simulink model "Senorless"  (R2023a)
settings: Solver=FixedStepDiscrete  StartTime=0.0  StopTime=2  FixedStep=1/FOC_FRQ  RelTol=1e-3
values from neighbouring files (symbols this model uses):
  ADC_REF = 3.6    [Senorless.sldd]
  ADC_SAMPLE_MAX = 32767.0    [Senorless.sldd]
  AMP_GAIN = 32.0    [Senorless.sldd]
  CURR_INPUT = 3276.0    [Senorless.sldd]
  CURR_KI = 380.0    [Senorless.sldd]
  CURR_KP = 0.04    [Senorless.sldd]
  CURR_LIMIT = 1.1    [Senorless.sldd]
  CURR_OVER = 34.0    [Senorless.sldd]
  CURR_POINT_GAIN = 7.0    [Senorless.sldd]
  CURR_STEP = 32760.0    [Senorless.sldd]
  CURR_UNDER = 0.03    [Senorless.sldd]
  CURR_WIDTH = 250.0    [Senorless.sldd]
  FOC_FRQ = 36000.0    [Senorless.sldd]
  GAMMA = 32767.0    [Senorless.sldd]
  HFI_ID = 2.125    [Senorless.sldd]
  IMAX = 34.0    [Senorless.sldd]
  LPF_FRQ = 300.0    [Senorless.sldd]
  MOTOR_DAMPER = 8.3E-7    [Senorless.sldd]
  MOTOR_FLUX = 0.0012713112    [Senorless.sldd]
  MOTOR_INERTIA = 1.02E-6    [Senorless.sldd]
  MOTOR_LS = 1.8E-5    [Senorless.sldd]
  MOTOR_PN = 7.0    [Senorless.sldd]
  MOTOR_RS = 0.065    [Senorless.sldd]
  NS_COMP_UD = 0.531    [Senorless.sldd]
  PLL_LIMIT = 0.95    [Senorless.sldd]
  PLL_WIDTH = 500.0    [Senorless.sldd]
  PWM_FRQ = 96000000.0    [Senorless.sldd]
  RS_HUNT = 0.002    [Senorless.sldd]
  SMOK_FRQ = 1200.0    [Senorless.sldd]
  SPD_LIMIT = 0.8    [Senorless.sldd]
  SPD_LPF_LEVEL = 15.0    [Senorless.sldd]
  SPD_MAX = 8100.0    [Senorless.sldd]
  SPD_MIN = -8100.0    [Senorless.sldd]
  SPD_REDUCE = 380.0    [Senorless.sldd]
  SPD_STEP = 3.0    [Senorless.sldd]
  SPD_WIDTH = 10.0    [Senorless.sldd]
  TS_POINT_GAIN = 10.0    [Senorless.sldd]
  UDC = 17.0    [Senorless.sldd]
  UDC_GAIN = 21.0    [Senorless.sldd]
  UDC_POINT_GAIN = 10.0    [Senorless.sldd]
undefined symbols (not defined in the file or in its folder): curr_q_ki, curr_q_kp, DiscIntNeverNeededParam, magnitude, PLL_LPF_LEVEL, Udc
libraries: simulink x20, slpidlib x5, mcbcontrolslib x4, mcbplantlib x1, autolibpmsminterior x1, autolibpmsmexterior x1, spspowerguiLib x1
(part 5 of 7)

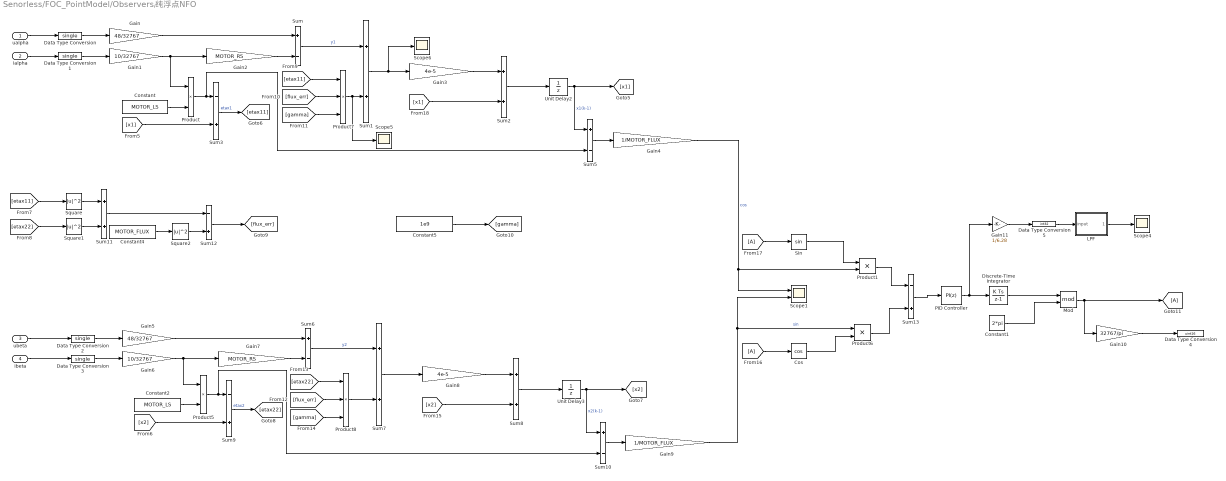
== system Senorless/FOC_PointModel/Observers/纯浮点NFO ==
  ualpha : Inport
  ialpha : Inport  Port=2
  ubeta : Inport  Port=3
  ibeta : Inport  Port=4
  Constant : Constant  Value=MOTOR_LS
  Constant1 : Constant  Value=2*pi  OutDataTypeStr=single
  Constant2 : Constant  Value=MOTOR_LS
  Constant4 : Constant  Value=MOTOR_FLUX
  Constant5 : Constant  Value=1e9  OutDataTypeStr=single
  Cos : Trigonometry  Operator=cos
  Data Type Conversion{,1..3} (4 alike) : DataTypeConversion  OutDataTypeStr=single  SaturateOnIntegerOverflow=off  RndMeth=Floor
  Data Type Conversion4 : DataTypeConversion  OutDataTypeStr=uint16  SaturateOnIntegerOverflow=off  RndMeth=Floor
  Data Type Conversion5 : DataTypeConversion  OutDataTypeStr=int32  SaturateOnIntegerOverflow=off  RndMeth=Floor
  Discrete-Time Integrator : DiscreteIntegrator  SampleTime=-1  ICPrevOutput=DiscIntNeverNeededParam  ICPrevScaledInput=DiscIntNeverNeededParam
  From16 : From
  From17 : From
  Gain : Gain  Gain=48/32767
  Gain1 : Gain  Gain=10/32767
  Gain10 : Gain  Gain=32767/pi
  Gain11 : Gain  Gain=1/6.28
  Gain2 : Gain  Gain=MOTOR_RS
  Gain3 : Gain  Gain=4e-5  OutDataTypeStr=single
  Gain4 : Gain  Gain=1/MOTOR_FLUX
  Gain5 : Gain  Gain=48/32767
  Gain6 : Gain  Gain=10/32767
  Gain7 : Gain  Gain=MOTOR_RS
  Gain8 : Gain  Gain=4e-5  OutDataTypeStr=single
  Gain9 : Gain  Gain=1/MOTOR_FLUX
  Goto11 : Goto
  LPF : Subsystem  TreatAsAtomicUnit=on
  Mod : Math  Operator=mod
  PID Controller : slpidlib/PID Controller  Controller=PI  Form=Parallel  TimeDomain=Discrete-time  UseExternalTs=off  SampleTime=-1  IntegratorMethod=Forward Euler  FilterMethod=Forward Euler  ControllerParametersSource=internal  P=2*800  I=800*800  UseKiTs=off  D=0  N=100  UseFilter=on  TunerSelectOption=Transfer Function Based (PID Tuner App)  InitialConditionSource=internal  InitialConditionForIntegrator=0  InitialConditionForFilter=0  DifferentiatorICPrevScaledInput=0  ExternalReset=none  TrackingMode=off  Kt=1  LimitOutput=off  SatLimitsSource=internal  UpperSaturationLimit=inf  LowerSaturationLimit=-inf  LinearizeAsGain=on  AntiWindupMode=none  Kb=1  LimitIntegrator=off  UpperIntegratorSaturationLimit=inf  LowerIntegratorSaturationLimit=-inf  POutMin=[]  POutMax=[]  IOutMin=[]  IOutMax=[]  DOutMin=[]  DOutMax=[]  NOutMin=[]  NOutMax=[]  SumOutMin=[]  SumOutMax=[]  SaturationOutMin=[]  SaturationOutMax=[]  PParamMin=[]  PParamMax=[]  IParamMin=[]  IParamMax=[]  DParamMin=[]  DParamMax=[]  NParamMin=[]  NParamMax=[]  KbParamMin=[]  KbParamMax=[]  KtParamMin=[]  KtParamMax=[]  KbOutMin=[]  KbOutMax=[]  KtOutMin=[]  KtOutMax=[]  IntegratorOutMin=[]  IntegratorOutMax=[]  FilterOutMin=[]  FilterOutMax=[]  SumI1OutMin=[]  SumI1OutMax=[]  SumI2OutMin=[]  SumI2OutMax=[]  SumI3OutMin=[]  SumI3OutMax=[]  SumI4OutMin=[]  SumI4OutMax=[]  SumDOutMin=[]  SumDOutMax=[]  DifferentiatorOutMin=[]  DifferentiatorOutMax=[]  FilterDiffOutCoefMin=[]  FilterDiffOutCoefMax=[]  ReciprocalOutMin=[]  ReciprocalOutMax=[]  SumDenOutMin=[]  SumDenOutMax=[]  SumNumOutMin=[]  SumNumOutMax=[]  DivideOutMin=[]  DivideOutMax=[]  UdiffTsProdOutMin=[]  UdiffTsProdOutMax=[]  NTsProdOutMin=[]  NTsProdOutMax=[]  UintegralTsProdOutMin=[]  UintegralTsProdOutMax=[]  UngainTsProdOutMin=[]  UngainTsProdOutMax=[]  ClampingZeroOutDataTypeStr=Inherit: Inherit via back propagation  ClampingZeroOutMin=[]  ClampingZeroOutMax=[]  FilterDenConstantOutDataTypeStr=Inherit: Inherit via back propagation  FilterDenConstantOutMin=[]  FilterDenConstantOutMax=[]  PCopyOutDataTypeStr=Inherit: Inherit via back propagation  PCopyOutMin=[]  PCopyOutMax=[]  NCopyOutDataTypeStr=Inherit: Inherit via back propagation  NCopyOutMin=[]  NCopyOutMax=[]  IntegratorContinuousStateAttributes=''  IntegratorStateMustResolveToSignalObject=off  IntegratorRTWStateStorageClass=Auto  FilterContinuousStateAttributes=''  FilterStateMustResolveToSignalObject=off  FilterRTWStateStorageClass=Auto  ParallelPVariant=InternalParameters  IdealPVariant=Disabled  IVariant=InternalParameters  DVariant=Disabled  IntegratorVariant=Discrete  SatVariant=Disabled  AWVariant=Passthrough  PCopyVariant=Disabled  TRVariant=Disabled  FdbkBlocksVariant=Forward  IdealPFdbkVariant=Disabled  SatFdbkVariant=Disabled  DerivativeFilterVariant=Disabled  NVariant=Disabled  NCopyVariant=Disabled_SignalSpec  FilterICVariant=Disabled  IntegratorICVariant=InternalICs  ExternalResetVariant=Disabled  TRSumVariant=Passthrough  SumFdbkVariant=Disabled  SumVariant=Sum_PI  TsampFilterVariant=InternalTs  TsampNgainVariant=Passthrough  TsampIntegralVariant=Disabled_SignalSpec  ExternalSaturationOutDataTypeStr=Inherit: Same as second input
  Product{,1,5..6} (4 alike) : Product
  Product7 : Product  Inputs=3
  Product8 : Product  Inputs=3
  Scope1 : Scope  NumInputPorts=2
  Scope4 : Scope
  Scope5 : Scope
  Scope6 : Scope
  Sin : Trigonometry
  Square : Math  Operator=magnitude^2  OutputSignalType=real
  Square1 : Math  Operator=magnitude^2  OutputSignalType=real
  Square2 : Math  Operator=magnitude^2  OutputSignalType=real
  Sum{,5..6,10} (4 alike) : Sum  Inputs=+-
  Sum{1..2,7..8,11} (5 alike) : Sum
  Sum{3,9,12..13} (4 alike) : Sum  Inputs=-+
  Unit Delay2 : UnitDelay  SampleTime=-1  HasFrameUpgradeWarning=on
  Unit Delay3 : UnitDelay  SampleTime=-1  HasFrameUpgradeWarning=on
  wires:
  Gain8/1 -> Sum8/1
  Constant2/1 -> Product5/2
  Sum/1 -> Sum1/1  "y1"
  Sum2/1 -> Unit Delay2/1
  Sum10/1 -> Gain9/1
  Gain4/1 -> Scope1/1, Product1/2  "cos"
  [x1] -> Sum2/2
  ibeta/1 -> Data Type Conversion3/1
  ubeta/1 -> Data Type Conversion2/1
  [etax22] -> Square1/1
  Data Type Conversion/1 -> Gain/1
  [etax11] -> Square/1
  Sum9/1 -> [etax22]  "etax2"
  Gain/1 -> Sum/1
  Product5/1 -> Sum10/2, Sum9/1
  Square2/1 -> Sum12/2
  Product1/1 -> Sum13/1
  Gain5/1 -> Sum6/1
  Sum1/1 -> Scope6/1, Gain3/1
  Data Type Conversion3/1 -> Gain6/1
  Sum8/1 -> Unit Delay3/1
  [flux_err] -> Product8/2
  Sum5/1 -> Gain4/1
  PID Controller/1 -> Gain11/1, Discrete-Time Integrator/1
  Cos/1 -> Product6/2
  [etax22] -> Product8/1
  [gamma] -> Product7/3
  Square1/1 -> Sum11/2
  [x1] -> Sum3/2
  Constant/1 -> Product/2
  Product7/1 -> Scope5/1, Sum1/2
  Sum13/1 -> PID Controller/1
  Square/1 -> Sum11/1
  Sum6/1 -> Sum7/1  "y2"
  Product8/1 -> Sum7/2
  Discrete-Time Integrator/1 -> Mod/1
  [flux_err] -> Product7/2
  Constant5/1 -> [gamma]
  Constant4/1 -> Square2/1
  Sum12/1 -> [flux_err]
  [gamma] -> Product8/3
  Sum3/1 -> [etax11]  "etax1"
  Gain9/1 -> Scope1/2, Product6/1  "sin"
  [etax11] -> Product7/1
  Gain7/1 -> Sum6/2
  Gain1/1 -> Product/1, Gain2/1
  Gain10/1 -> Data Type Conversion4/1
  ialpha/1 -> Data Type Conversion1/1
  Gain6/1 -> Gain7/1, Product5/1
  Gain3/1 -> Sum2/1
  Sin/1 -> Product1/1
  Product6/1 -> Sum13/2
  Sum11/1 -> Sum12/1
  From17/1 -> Sin/1
  Data Type Conversion1/1 -> Gain1/1
  Gain11/1 -> Data Type Conversion5/1
  Mod/1 -> Gain10/1, Goto11/1
  From16/1 -> Cos/1
  Constant1/1 -> Mod/2
  [x2] -> Sum8/2
  Gain2/1 -> Sum/2
  [x2] -> Sum9/2
  Data Type Conversion2/1 -> Gain5/1
  Sum7/1 -> Gain8/1
  Unit Delay3/1 -> Sum10/1, [x2]  "x2(k-1)"
  Unit Delay2/1 -> Sum5/1, [x1]  "x1(k-1)"
  Product/1 -> Sum5/2, Sum3/1
  LPF/1(output) -> Scope4/1
  Data Type Conversion5/1 -> LPF/1(input)
  ualpha/1 -> Data Type Conversion/1

== system Senorless/FOC_PointModel/Park/滤波器 ==
  input : Inport
  Constant13 : Constant  Value=2*pi*250  OutDataTypeStr=int32
  Gain : Gain  Gain=1.414*32767  ParamDataTypeStr=int32  OutDataTypeStr=int32  RndMeth=Zero
  Gain1 : Gain  Gain=0.707*32767  ParamDataTypeStr=int32  OutDataTypeStr=int32  RndMeth=Zero
  Product : Product  OutDataTypeStr=int32  RndMeth=Zero
  Product1 : Product  OutDataTypeStr=int32  RndMeth=Zero
  Scope : Scope  NumInputPorts=2
  Shift Arithmetic : ArithShift  BitShiftNumber=15
  Shift Arithmetic1 : ArithShift  BitShiftNumber=15
  Sum5 : Sum  Inputs=-+|  AccumDataTypeStr=int32  OutDataTypeStr=int32  RndMeth=Zero
  Sum8 : Sum  Inputs=|+-  AccumDataTypeStr=int32  OutDataTypeStr=int32  RndMeth=Zero
  Unit Delay : UnitDelay  SampleTime=-1  HasFrameUpgradeWarning=on
  input1 : InportShadow
  积分器4 : Subsystem
      settings: MinAlgLoopOccurrences=on
  积分器5 : Subsystem
      settings: MinAlgLoopOccurrences=on
  output : Outport
  wires:
  Constant13/1 -> Product/2, Product1/1
  Product/1 -> 积分器4/1(input)
  Product1/1 -> 积分器5/1(input)
  Sum8/1 -> Product/1
  input1/1 -> Scope/2
  积分器4/1(output) -> Unit Delay/1
  Unit Delay/1 -> Sum5/1, Product1/2
  Gain/1 -> Shift Arithmetic/1
  Gain1/1 -> Shift Arithmetic1/1
  积分器5/1(output) -> Gain1/1, Sum8/2
  Shift Arithmetic1/1 -> Scope/1, output/1
  input/1 -> Sum5/2
  Sum5/1 -> Gain/1
  Shift Arithmetic/1 -> Sum8/1

== system Senorless/FOC_PointModel/SVPWM/AntiClark ==
  note: Va = Valpha;
      | Vb = Valpha*(-1/2)+Vbeta*sqrt(3)/2
      | Vc = Valpha*(-1/2)-Vbeta*sqrt(3)/2
  Valpha : Inport
  Vbeta : Inport  Port=2
  Gain1 : Gain  Gain=32767*sqrt(3)/2  ParamDataTypeStr=int16  OutDataTypeStr=int32  RndMeth=Zero
  Shift Arithmetic : ArithShift  BitShiftNumber=15
  Shift Arithmetic1 : ArithShift  BitShiftNumber=1
  Sum : Sum  Inputs=|-+  RndMeth=Zero
  Sum1 : Sum  Inputs=--|  RndMeth=Zero
  Va : Outport
  Vb : Outport  Port=2
  Vc : Outport  Port=3
  wires:
  Vbeta/1 -> Gain1/1
  Shift Arithmetic1/1 -> Sum1/2, Sum/1
  Sum/1 -> Vb/1
  Gain1/1 -> Shift Arithmetic/1
  Sum1/1 -> Vc/1
  Shift Arithmetic/1 -> Sum1/1, Sum/2
  Valpha/1 -> Va/1, Shift Arithmetic1/1

== system Senorless/FOC_PointModel/SVPWM/ei_t ==
  note: V0 = -1/2(Vmax+Vmin)
  Vabc : Inport
  Min : MinMax  RndMeth=Zero
  Min1 : MinMax  Function=max  RndMeth=Zero
  Shift Arithmetic : ArithShift  BitShiftNumber=1
  Sum : Sum  OutDataTypeStr=int32  RndMeth=Zero
  Unary Minus : UnaryMinus
  ei_t : Outport
  wires:
  Min/1 -> Sum/1
  Sum/1 -> Shift Arithmetic/1
  Min1/1 -> Sum/2
  Shift Arithmetic/1 -> Unary Minus/1
  Unary Minus/1 -> ei_t/1
  Vabc/1 -> Min1/1, Min/1

== system Senorless/FOC_PointModel/idq_Controller/PI Controller ==
  input : Inport
  Kp : Inport  Port=2
  Ki : Inport  Port=3
  Data Store Read3 : DataStoreRead  DataStoreName=Curr_Limit  IndexOptions=Index vector (dialog)  Indices=1  OutputSizes=1
  Gain : Gain  Gain=-1  OutDataTypeStr=int32  RndMeth=Zero
  Product2 : Product  OutDataTypeStr=int32  RndMeth=Zero
  Saturation Dynamic2 : simulink/Discontinuities/Saturation Dynamic  OutMin=[]  OutMax=[]  OutDataTypeStr=Inherit: Same as second input  OutDataType=fixdt(1, 16)  OutScaling=2^-10  RndMeth=Zero  DoSatur=off
  Scope : Scope  NumInputPorts=2
  Sum : Sum  OutDataTypeStr=int32  RndMeth=Zero
  input1 : InportShadow
  积分器 : Subsystem
      settings: MinAlgLoopOccurrences=on
  output : Outport  OutputWhenDisabled=reset  InitialOutput=int32(0)
  wires:
  input/1 -> Product2/1
  Kp/1 -> Product2/2
  Ki/1 -> 积分器/1(Ki)
  input1/1 -> 积分器/2(input)
  Product2/1 -> Scope/1, Sum/1
  积分器/1(output) -> Sum/2, Scope/2
  Sum/1 -> Saturation Dynamic2/2
  Saturation Dynamic2/1 -> output/1
  Data Store Read3/1 -> [limit]
  [limit] -> Gain/1
  Gain/1 -> Saturation Dynamic2/3
  [limit] -> Saturation Dynamic2/1

== system Senorless/FOC_PointModel/idq_Controller/PI Controller1 ==
  Ki : Inport
  Kp : Inport  Port=2
  input : Inport  Port=3
  Data Store Read3 : DataStoreRead  DataStoreName=Curr_Limit  IndexOptions=Index vector (dialog)  Indices=1  OutputSizes=1
  Gain : Gain  Gain=-1  OutDataTypeStr=int32  RndMeth=Zero
  Product2 : Product  OutDataTypeStr=int32  RndMeth=Zero
  Saturation Dynamic2 : simulink/Discontinuities/Saturation Dynamic  OutMin=[]  OutMax=[]  OutDataTypeStr=Inherit: Same as second input  OutDataType=fixdt(1, 16)  OutScaling=2^-10  RndMeth=Zero  DoSatur=off
  Scope : Scope  NumInputPorts=2
  Sum : Sum  OutDataTypeStr=int32  RndMeth=Zero
  input1 : InportShadow  Port=3
  积分器 : Subsystem
      settings: MinAlgLoopOccurrences=on
  output : Outport  OutputWhenDisabled=reset  InitialOutput=int32(0)
  wires:
  [limit] -> Saturation Dynamic2/1
  Gain/1 -> Saturation Dynamic2/3
  [limit] -> Gain/1
  Data Store Read3/1 -> [limit]
  Sum/1 -> Saturation Dynamic2/2
  积分器/1(output) -> Scope/2, Sum/2
  Product2/1 -> Sum/1, Scope/1
  input1/1 -> 积分器/2(input)
  Ki/1 -> 积分器/1(Ki)
  Kp/1 -> Product2/2
  input/1 -> Product2/1
  Saturation Dynamic2/1 -> output/1

== system Senorless/FOC_PointModel/idq_Controller/PI Controller2 ==
  input : Inport
  Kp : Inport  Port=2
  Ki : Inport  Port=3
  Reset : Inport  Port=4
  Xo : Inport  Port=5
  Action Port : ActionPort  InitializeStates=reset  ActionPortLabel=if(u1 > 0)
  Data Store Read3 : DataStoreRead  DataStoreName=Curr_Limit  IndexOptions=Index vector (dialog)  Indices=1  OutputSizes=1
  Gain : Gain  Gain=-1  OutDataTypeStr=int32  RndMeth=Zero
  MATLAB Function : MATLAB Function  TreatAsAtomicUnit=on
  Product2 : Product  OutDataTypeStr=int32  RndMeth=Zero
  Scope : Scope  NumInputPorts=2
  Sum : Sum  OutDataTypeStr=int32  RndMeth=Zero
  input1 : InportShadow
  积分器/双边沿初始化 : Subsystem
      settings: MinAlgLoopOccurrences=on
  output : Outport
  wires:
  [limit] -> MATLAB Function/2(up), Gain/1
  Gain/1 -> MATLAB Function/3(low)
  Data Store Read3/1 -> [limit]
  MATLAB Function/1(out) -> output/1
  Sum/1 -> MATLAB Function/1(in)
  积分器/双边沿初始化/1(output) -> Scope/2, Sum/2
  Product2/1 -> Sum/1, Scope/1
  input1/1 -> 积分器/双边沿初始化/2(input)
  Reset/1 -> 积分器/双边沿初始化/4(Reset)
  Xo/1 -> 积分器/双边沿初始化/3(Xo)
  Ki/1 -> 积分器/双边沿初始化/1(Ki)
  Kp/1 -> Product2/2
  input/1 -> Product2/1

== system Senorless/FOC_PointModel/idq_Controller/Subsystem ==
  Ud : Inport
  Uq : Inport  Port=2
  Constant : Constant  Value=16384*0.9  OutDataTypeStr=int16
  Data Type Conversion5 : DataTypeConversion  OutDataTypeStr=int16  SaturateOnIntegerOverflow=off
  Data Type Conversion6 : DataTypeConversion  OutDataTypeStr=int16  SaturateOnIntegerOverflow=off
  Scope : Scope
  Shift Arithmetic7 : ArithShift  BitShiftNumber=-0
  Sqrt1 : Sqrt  OutputSignalType=real  OutDataTypeStr=int16  RndMeth=Zero  IntermediateResultsDataTypeStr=int32
  Square2 : Math  Operator=square  OutputSignalType=real  OutDataTypeStr=int32  RndMeth=Zero
      settings: LockScale=on
  Square3 : Math  Operator=square  OutDataTypeStr=int32  RndMeth=Zero
      settings: LockScale=on
  Sum11 : Sum  AccumDataTypeStr=int32  OutDataTypeStr=int32
  Sum12 : Sum  Inputs=|-+
  Unit Delay5 : UnitDelay  SampleTime=-1  HasFrameUpgradeWarning=on
  Wrap To Zero1 : simulink/Discontinuities/Wrap To Zero  Threshold=int16(0)
  -Id : Outport
  wires:
  Data Type Conversion5/1 -> Square2/1
  Wrap To Zero1/1 -> Shift Arithmetic7/1
  Sum11/1 -> Sqrt1/1
  Sqrt1/1 -> Scope/1, Sum12/1
  Data Type Conversion6/1 -> Square3/1
  Square2/1 -> Sum11/1
  Sum12/1 -> Wrap To Zero1/1
  Constant/1 -> Sum12/2
  Uq/1 -> Data Type Conversion6/1
  Square3/1 -> Sum11/2
  Ud/1 -> Data Type Conversion5/1
  Shift Arithmetic7/1 -> Unit Delay5/1
  Unit Delay5/1 -> -Id/1

== system Senorless/FOC_PointModel/标志位/积分器 ==
  input : Inport
  Xo : Inport  Port=2
  Constant : Constant  OutDataTypeStr=int16
  Data Store Read1 : DataStoreRead  DataStoreName=Ts_Point  IndexOptions=Index vector (dialog)  Indices=1  OutputSizes=1
  Delay : Delay  DelayLength=1  InitialConditionSource=Input port
      settings: InputPortMap=u0,p4
  Product1 : Product  OutDataTypeStr=int32  RndMeth=Zero
  Product2 : Product  OutDataTypeStr=int32  RndMeth=Zero
  Shift Arithmetic : ArithShift  BitShiftNumberSource=Input port  BitShiftNumber=8  BitShiftDirection=Right
      settings: InputPortMap=u0,p1
  Sum : Sum  Inputs=|++  OutDataTypeStr=int32  RndMeth=Zero
  周期定点化适当放大2^n : Constant  Value=TS_POINT_GAIN
  这个是缩小周期增益的 : ArithShift  BitShiftNumber=15  DiagnosticForOORShift=Error
  output : Outport
  wires:
  Sum/1 -> Delay/1, output/1
  Product2/1 -> 这个是缩小周期增益的/1
  input/1 -> Shift Arithmetic/1
  Data Store Read1/1 -> Product2/1
  Shift Arithmetic/1 -> Product2/2
  周期定点化适当放大2^n/1 -> Shift Arithmetic/2
  Xo/1 -> Delay/2
  这个是缩小周期增益的/1 -> Product1/1
  Constant/1 -> Product1/2
  Product1/1 -> Sum/1
  Delay/1 -> Sum/2

== system Senorless/FOC_PointModel/观测器闭环//速度环/PI Controller ==
  input : Inport
  Ki : Inport  Port=2
  Kp : Inport  Port=3
  init : Inport  Port=4
  Data Store Read3 : DataStoreRead  DataStoreName=Speed_Limit  IndexOptions=Index vector (dialog)  Indices=1  OutputSizes=1
  Gain : Gain  Gain=-1  OutDataTypeStr=int32  RndMeth=Zero
  Product2 : Product  OutDataTypeStr=int32  RndMeth=Zero
  Saturation Dynamic2 : simulink/Discontinuities/Saturation Dynamic  OutMin=[]  OutMax=[]  OutDataTypeStr=Inherit: Same as second input  OutDataType=fixdt(1, 16)  OutScaling=2^-10  RndMeth=Zero  DoSatur=off
  Scope : Scope  NumInputPorts=2
  Scope1 : Scope  NumInputPorts=2
  Scope2 : Scope
  Sum : Sum  OutDataTypeStr=int32  RndMeth=Zero
  input1 : InportShadow
  积分器1 : Subsystem
      settings: MinAlgLoopOccurrences=on
  output : Outport
  wires:
  Sum/1 -> Saturation Dynamic2/2
  Data Store Read3/1 -> [limit]
  Product2/1 -> Sum/1, Scope/1, Scope1/2
  积分器1/1(output) -> Sum/2, Scope/2
  Ki/1 -> 积分器1/1(Ki)
  Gain/1 -> Saturation Dynamic2/3
  [limit] -> Saturation Dynamic2/1
  [limit] -> Gain/1
  Saturation Dynamic2/1 -> output/1
  input1/1 -> 积分器1/2(input)
  input/1 -> Scope1/1, Product2/1
  Kp/1 -> Scope2/1, Product2/2
  init/1 -> 积分器1/3(init)

== system Senorless/FOC_PointModel/Err/闭环错误判断/SUM ==
  in : Inport
  Action Port : ActionPort  InitializeStates=reset  ActionPortLabel=if(u1 > 0)
  Sum : Sum  Inputs=|++  OutDataTypeStr=int32  RndMeth=Zero
  Unit Delay2 : UnitDelay  SampleTime=-1  HasFrameUpgradeWarning=on
  out : Outport
  wires:
  Sum/1 -> Unit Delay2/1
  in/1 -> Sum/1
  Unit Delay2/1 -> out/1, Sum/2

== system Senorless/FOC_PointModel/Err/闭环错误判断/ZERO ==
  Action Port : ActionPort  InitializeStates=reset  ActionPortLabel=else
  Constant : Constant  Value=0  OutDataTypeStr=int32
  out : Outport
  wires:
  Constant/1 -> out/1

== system Senorless/FOC_PointModel/NS辨识/加速积分角度/积分器 ==
  K_p : Inport
  input : Inport  Port=2
  Xo : Inport  Port=3
  Reset : Inport  Port=4
  Data Store Memory : DataStoreMemory  DataStoreName=tmp  WriteAfterWriteMsg=warning  ShowAdditionalParam=off
  Data Store Read : DataStoreRead  DataStoreName=tmp  IndexOptions=Index vector (dialog)  Indices=1  OutputSizes=1
  Data Store Write : DataStoreWrite  DataStoreName=tmp  IndexOptions=Index vector (dialog)  Indices=1  OutputSizes=1
  Data Type Conversion2 : DataTypeConversion  OutDataTypeStr=int32  SaturateOnIntegerOverflow=off
  Data Type Conversion3 : DataTypeConversion  OutDataTypeStr=int32  SaturateOnIntegerOverflow=off
  Divide : Product  Inputs=*/  OutDataTypeStr=int32  RndMeth=Zero
  Product : Product  OutDataTypeStr=int64  RndMeth=Zero
  Product1 : Product  OutDataTypeStr=int64  RndMeth=Zero
  Reset_Block : Subsystem
  Sum : Sum  Inputs=|++  OutDataTypeStr=int64  RndMeth=Zero
  Unit Delay : UnitDelay  SampleTime=-1  HasFrameUpgradeWarning=on
  积分器运行频率 : Constant  Value=FOC_FRQ
  output : Outport
  wires:
  K_p/1 -> Product1/1, Product/2
  Reset/1 -> Reset_Block/Trigger
  Data Store Read/1 -> Sum/2
  Unit Delay/1 -> Data Store Write/1
  Product/1 -> Reset_Block/1(Xo)
  Divide/1 -> Product1/2
  input/1 -> Divide/1
  Product1/1 -> Sum/1
  积分器运行频率/1 -> Data Type Conversion3/1
  Data Type Conversion3/1 -> Divide/2
  Xo/1 -> Data Type Conversion2/1
  Data Type Conversion2/1 -> Product/1
  Sum/1 -> Unit Delay/1, output/1

== system Senorless/FOC_PointModel/NS辨识/加速积分角度/积分器2 ==
  note: 此处相减作用是与后面的++相抵消，这样初始化后第一个输出值就是reset值，不然是reset值+Kp*input值
  K_p : Inport
  input : Inport  Port=2
  Xo : Inport  Port=3
  Reset : Inport  Port=4
  Data Store Memory : DataStoreMemory  DataStoreName=tmp  WriteAfterWriteMsg=warning  ShowAdditionalParam=off
  Data Store Read : DataStoreRead  DataStoreName=tmp  IndexOptions=Index vector (dialog)  Indices=1  OutputSizes=1
  Data Store Write : DataStoreWrite  DataStoreName=tmp  IndexOptions=Index vector (dialog)  Indices=1  OutputSizes=1
  Data Type Conversion2 : DataTypeConversion  OutDataTypeStr=int32  SaturateOnIntegerOverflow=off
  Data Type Conversion3 : DataTypeConversion  OutDataTypeStr=int32  SaturateOnIntegerOverflow=off
  Divide : Product  Inputs=*/  OutDataTypeStr=int32  RndMeth=Zero
  Product : Product  OutDataTypeStr=int64  RndMeth=Zero
  Product1 : Product  OutDataTypeStr=int64  RndMeth=Zero
  Reset_Block : Subsystem
  Sum : Sum  Inputs=|++  OutDataTypeStr=int64  RndMeth=Zero
  Sum1 : Sum  Inputs=|+-  OutDataTypeStr=int64  RndMeth=Zero
  Unit Delay : UnitDelay  SampleTime=-1  HasFrameUpgradeWarning=on
  积分器运行频率 : Constant  Value=FOC_FRQ
  output : Outport
  wires:
  K_p/1 -> Product1/1, Product/2
  Reset/1 -> Reset_Block/Trigger
  Data Store Read/1 -> Sum/2
  Sum/1 -> Unit Delay/1, output/1
  Unit Delay/1 -> Data Store Write/1
  Product/1 -> Sum1/1
  Divide/1 -> Product1/2
  input/1 -> Divide/1
  Product1/1 -> Sum1/2, Sum/1
  积分器运行频率/1 -> Data Type Conversion3/1
  Data Type Conversion3/1 -> Divide/2
  Xo/1 -> Data Type Conversion2/1
  Data Type Conversion2/1 -> Product/1
  Sum1/1 -> Reset_Block/1(Xo)

== system Senorless/FOC_PointModel/NS辨识/加速积分角度/积分器3 ==
  input : Inport
  Constant : Constant  OutDataTypeStr=int16
  Data Store Read1 : DataStoreRead  DataStoreName=Ts_Point  IndexOptions=Index vector (dialog)  Indices=1  OutputSizes=1
  Product1 : Product  OutDataTypeStr=int32  RndMeth=Zero
  Product2 : Product  OutDataTypeStr=int32  RndMeth=Zero
  Shift Arithmetic : ArithShift  BitShiftNumberSource=Input port  BitShiftNumber=8  BitShiftDirection=Right
      settings: InputPortMap=u0,p1
  Sum : Sum  Inputs=++|  OutDataTypeStr=int32  RndMeth=Zero
  Unit Delay : UnitDelay  SampleTime=-1  HasFrameUpgradeWarning=on
  周期定点化适当放大2^n : Constant  Value=TS_POINT_GAIN
  这个是缩小周期增益的 : ArithShift  BitShiftNumber=15  DiagnosticForOORShift=Error
  output : Outport
  wires:
  周期定点化适当放大2^n/1 -> Shift Arithmetic/2
  Shift Arithmetic/1 -> Product2/2
  Data Store Read1/1 -> Product2/1
  input/1 -> Shift Arithmetic/1
  Product2/1 -> 这个是缩小周期增益的/1
  Sum/1 -> Unit Delay/1, output/1
  这个是缩小周期增益的/1 -> Product1/1
  Constant/1 -> Product1/2
  Product1/1 -> Sum/2
  Unit Delay/1 -> Sum/1

== system Senorless/FOC_PointModel/NS辨识/加速积分角度/积分器4 ==
  input : Inport
  Constant : Constant  OutDataTypeStr=int16
  Data Store Read1 : DataStoreRead  DataStoreName=Ts_Point  IndexOptions=Index vector (dialog)  Indices=1  OutputSizes=1
  Product1 : Product  OutDataTypeStr=int32  RndMeth=Zero
  Product2 : Product  OutDataTypeStr=int32  RndMeth=Zero
  Shift Arithmetic : ArithShift  BitShiftNumberSource=Input port  BitShiftNumber=8  BitShiftDirection=Right
      settings: InputPortMap=u0,p1
  Sum : Sum  Inputs=++|  OutDataTypeStr=int32  RndMeth=Zero
  Unit Delay : UnitDelay  SampleTime=-1  HasFrameUpgradeWarning=on
  周期定点化适当放大2^n : Constant  Value=TS_POINT_GAIN
  这个是缩小周期增益的 : ArithShift  BitShiftNumber=15  DiagnosticForOORShift=Error
  output : Outport
  wires:
  Unit Delay/1 -> Sum/1
  Product1/1 -> Sum/2
  Constant/1 -> Product1/2
  这个是缩小周期增益的/1 -> Product1/1
  Sum/1 -> output/1, Unit Delay/1
  Product2/1 -> 这个是缩小周期增益的/1
  input/1 -> Shift Arithmetic/1
  Data Store Read1/1 -> Product2/1
  Shift Arithmetic/1 -> Product2/2
  周期定点化适当放大2^n/1 -> Shift Arithmetic/2

== system Senorless/FOC_PointModel/Observers/PLL/PI Controller ==
  input : Inport
  Kp : Inport  Port=2
  Ki : Inport  Port=3
  Data Store Read3 : DataStoreRead  DataStoreName=PLL_Limit  IndexOptions=Index vector (dialog)  Indices=1  OutputSizes=1
  Gain : Gain  Gain=-1  OutDataTypeStr=int32  RndMeth=Zero
  Product2 : Product  OutDataTypeStr=int32  RndMeth=Zero
  Saturation Dynamic2 : simulink/Discontinuities/Saturation Dynamic  OutMin=[]  OutMax=[]  OutDataTypeStr=Inherit: Same as second input  OutDataType=fixdt(1, 16)  OutScaling=2^-10  RndMeth=Zero  DoSatur=off
  Scope : Scope  NumInputPorts=2
  Sum : Sum  OutDataTypeStr=int32  RndMeth=Zero
  input1 : InportShadow
  积分器 : Subsystem
      settings: MinAlgLoopOccurrences=on
  output : Outport
  wires:
  input/1 -> Product2/1
  Kp/1 -> Product2/2
  Ki/1 -> 积分器/1(Ki)
  input1/1 -> 积分器/2(input)
  Product2/1 -> Sum/1, Scope/1
  积分器/1(output) -> Scope/2, Sum/2
  Data Store Read3/1 -> [Limit]
  [Limit] -> Gain/1
  Gain/1 -> Saturation Dynamic2/3
  Sum/1 -> Saturation Dynamic2/2
  [Limit] -> Saturation Dynamic2/1
  Saturation Dynamic2/1 -> output/1

== system Senorless/FOC_PointModel/Observers/PLL/sincos_4096 ==
  theta : Inport
  Constant1 : Constant  Value=128  OutDataTypeStr=uint16
  Constant3 : Constant  Value=16384+128  OutDataTypeStr=uint16
  Shift Arithmetic : ArithShift  BitShiftNumber=4
  Shift Arithmetic1 : ArithShift  BitShiftNumber=4
  Sin : Lookup_n-D  NumberOfTableDimensions=1  BreakpointsSpecification=Even spacing  BreakpointsForDimension1=uint16(linspace(0,511,512))  BreakpointsForDimension1DataTypeStr=uint16  IndexSearchMethod=Linear search  BeginIndexSearchUsingPreviousIndexResult=on  UseOneInputPortForAllInputData=on  Table=int16(32767*sin(linspace(0,2*pi,4096)))  TableDataTypeStr=int16  IntermediateResultsDataTypeStr=int32  InterpMethod=Flat  ExtrapMethod=Clip  RemoveProtectionInput=on  ApplyFullPrecisionForLinearInterpolation=on  InternalRulePriority=Speed  OutDataTypeStr=int16  RndMeth=Zero  FractionDataTypeStr=fixdt(1,16,0)  InputSameDT=off
  Sin1 : Lookup_n-D  NumberOfTableDimensions=1  BreakpointsSpecification=Even spacing  BreakpointsForDimension1=uint16(linspace(0,511,512))  BreakpointsForDimension1DataTypeStr=uint16  IndexSearchMethod=Linear search  BeginIndexSearchUsingPreviousIndexResult=on  UseOneInputPortForAllInputData=on  Table=int16(32767*sin(linspace(0,2*pi,4096)))  TableDataTypeStr=int16  IntermediateResultsDataTypeStr=int32  InterpMethod=Flat  ExtrapMethod=Clip  RemoveProtectionInput=on  ApplyFullPrecisionForLinearInterpolation=on  InternalRulePriority=Speed  OutDataTypeStr=int16  RndMeth=Zero  FractionDataTypeStr=fixdt(1,16,0)  InputSameDT=off
  Sin2 : Lookup_n-D  Commented=on  NumberOfTableDimensions=1  BreakpointsSpecification=Even spacing  BreakpointsForDimension1=uint16(linspace(0,511,512))  BreakpointsForDimension1DataTypeStr=uint16  IndexSearchMethod=Linear search  BeginIndexSearchUsingPreviousIndexResult=on  UseOneInputPortForAllInputData=on  Table=|  TableDataTypeStr=int16  IntermediateResultsDataTypeStr=int32  InterpMethod=Flat  ExtrapMethod=Clip  RemoveProtectionInput=on  ApplyFullPrecisionForLinearInterpolation=on  InternalRulePriority=Speed  OutDataTypeStr=int16  RndMeth=Zero  FractionDataTypeStr=fixdt(1,16,0)  InputSameDT=off
      | int16([
      |  0 ,   402 ,   804 ,  1207 ,  1609 , ...
      |       2011 ,  2412 ,  2814 ,  3214 ,  3615 , ...
      |       4015 ,  4414 ,  4812 ,  5210 ,  5607 , ...
      |       6003 ,  6398 ,  6793 ,  7186 ,  7578 , ...
      |       7969 ,  8359 ,  8747 ,  9135 ,  9521 , ...
      |       9905 , 10288 , 10669 , 11049 , 11427 , ...
      |      11804 , 12178 , 12551 , 12922 , 13291 , ...
      |      13658 , 14022 , 14385 , 14746 , 15104 , ...
      |      15460 , 15814 , 16165 , 16514 , 16860 , ...
      |      17204 , 17546 , 17884 , 18220 , 18553 , ...
      |      18884 , 19211 , 19536 , 19857 , 20176 , ...
      |      20492 , 20804 , 21114 , 21420 , 21723 , ...
      |      22023 , 22319 , 22612 , 22902 , 23188 , ...
      |      23470 , 23750 , 24025 , 24297 , 24565 , ...
      |      24830 , 25090 , 25347 , 25601 , 25850 , ...
      |      26095 , 26337 , 26574 , 26808 , 27037 , ...
      |      27263 , 27484 , 27701 , 27914 , 28123 , ...
      |      28327 , 28527 , 28723 , 28915 , 29102 , ...
      |      29285 , 29463 , 29637 , 29806 , 29971 , ...
      |      30132 , 30288 , 30439 , 30586 , 30728 , ...
      |      30865 , 30998 , 31126 , 31250 , 31368 , ...
      |      31482 , 31592 , 31696 , 31796 , 31891 , ...
      |      31981 , 32066 , 32146 , 32222 , 32293 , ...
      |      32359 , 32419 , 32476 , 32527 , 32573 , ...
      |      32614 , 32651 , 32682 , 32709 , 32730 , ...
      |      32747 , 32759 , 32766 , 32767 , 32764 , ...
      |      32756 , 32743 , 32725 , 32703 , 32675 , ...
      |      32642 , 32604 , 32562 , 32514 , 32462 , ...
      |      32405 , 32343 , 32275 , 32204 , 32127 , ...
      |      32045 , 31959 , 31867 , 31771 , 31670 , ...
      |      31565 , 31454 , 31339 , 31219 , 31095 , ...
      |      30965 , 30831 , 30693 , 30549 , 30402 , ...
      |      30249 , 30092 , 29930 , 29764 , 29594 , ...
      |      29419 , 29239 , 29055 , 28867 , 28674 , ...
      |      28478 , 28276 , 28071 , 27861 , 27647 , ...
      |      27429 , 27207 , 26980 , 26750 , 26515 , ...
      |      26277 , 26034 , 25788 , 25538 , 25284 , ...
      |      25026 , 24764 , 24498 , 24229 , 23956 , ...
      |      23680 , 23400 , 23117 , 22830 , 22539 , ...
      |      22245 , 21948 , 21647 , 21344 , 21037 , ...
      |      20726 , 20413 , 20097 , 19777 , 19455 , ...
      |      19130 , 18801 , 18470 , 18136 , 17800 , ...
      |      17461 , 17119 , 16774 , 16427 , 16078 , ...
      |      15726 , 15371 , 15015 , 14656 , 14295 , ...
      |      13931 , 13566 , 13199 , 12829 , 12458 , ...
      |      12085 , 11710 , 11333 , 10954 , 10574 , ...
      |      10192 ,  9809 ,  9424 ,  9038 ,  8650 , ...
      |       8262 ,  7871 ,  7480 ,  7088 ,  6694 , ...
      |       6300 ,  5904 ,  5508 ,  5111 ,  4713 , ...
      |       4314 ,  3915 ,  3515 ,  3114 ,  2713 , ...
      |       2312 ,  1910 ,  1508 ,  1106 ,   704 , ...
      |        301 ,  -100 ,  -503 ,  -905 , -1307 , ...
      |      -1709 , -2111 , -2513 , -2914 , -3315 , ...
      |      -3715 , -4114 , -4513 , -4912 , -5309 , ...
      |      -5706 , -6102 , -6497 , -6891 , -7284 , ...
      |      -7676 , -8067 , -8456 , -8844 , -9231 , ...
      |      -9617 ,-10001 ,-10383 ,-10764 ,-11144 , ...
      |     -11521 ,-11897 ,-12271 ,-12644 ,-13014 , ...
      |     -13383 ,-13749 ,-14113 ,-14475 ,-14835 , ...
      |     -15193 ,-15549 ,-15902 ,-16253 ,-16601 , ...
      |     -16947 ,-17290 ,-17630 ,-17968 ,-18304 , ...
      |     -18636 ,-18966 ,-19293 ,-19616 ,-19937 , ...
      |     -20255 ,-20570 ,-20882 ,-21191 ,-21496 , ...
      |     -21798 ,-22097 ,-22393 ,-22685 ,-22973 , ...
      |     -23259 ,-23541 ,-23819 ,-24093 ,-24364 , ...
      |     -24632 ,-24895 ,-25155 ,-25411 ,-25663 , ...
      |     -25912 ,-26156 ,-26397 ,-26633 ,-26866 , ...
      |     -27094 ,-27318 ,-27538 ,-27755 ,-27966 , ...
      |     -28174 ,-28377 ,-28577 ,-28771 ,-28962 , ...
      |     -29148 ,-29330 ,-29507 ,-29680 ,-29848 , ...
      |     -30012 ,-30171 ,-30326 ,-30476 ,-30622 , ...
      |     -30763 ,-30899 ,-31031 ,-31157 ,-31280 , ...
      |     -31397 ,-31510 ,-31618 ,-31721 ,-31820 , ...
      |     -31914 ,-32003 ,-32087 ,-32166 ,-32240 , ...
      |     -32310 ,-32374 ,-32434 ,-32489 ,-32539 , ...
      |     -32584 ,-32624 ,-32659 ,-32689 ,-32715 , ...
      |     -32735 ,-32750 ,-32761 ,-32767 ,-32767 , ...
      |     -32763 ,-32754 ,-32739 ,-32720 ,-32696 , ...
      |     -32667 ,-32633 ,-32594 ,-32550 ,-32502 , ...
      |     -32448 ,-32390 ,-32326 ,-32258 ,-32185 , ...
      |     -32107 ,-32024 ,-31936 ,-31844 ,-31747 , ...
      |     -31644 ,-31538 ,-31426 ,-31310 ,-31189 , ...
      |     -31063 ,-30932 ,-30797 ,-30657 ,-30513 , ...
      |     -30364 ,-30210 ,-30052 ,-29889 ,-29722 , ...
      |     -29550 ,-29374 ,-29194 ,-29009 ,-28819 , ...
      |     -28626 ,-28428 ,-28225 ,-28019 ,-27808 , ...
      |     -27593 ,-27374 ,-27150 ,-26923 ,-26692 , ...
      |     -26456 ,-26217 ,-25973 ,-25726 ,-25475 , ...
      |     -25219 ,-24961 ,-24698 ,-24432 ,-24161 , ...
      |     -23888 ,-23610 ,-23330 ,-23045 ,-22757 , ...
      |     -22466 ,-22171 ,-21873 ,-21572 ,-21267 , ...
      |     -20959 ,-20648 ,-20334 ,-20017 ,-19697 , ...
      |     -19374 ,-19048 ,-18719 ,-18387 ,-18052 , ...
      |     -17715 ,-17375 ,-17033 ,-16688 ,-16340 , ...
      |     -15990 ,-15637 ,-15282 ,-14925 ,-14566 , ...
      |     -14204 ,-13840 ,-13474 ,-13106 ,-12737 , ...
      |     -12365 ,-11991 ,-11616 ,-11238 ,-10859 , ...
      |     -10479 ,-10097 , -9713 , -9328 , -8941 , ...
      |      -8553 , -8164 , -7774 , -7382 , -6989 , ...
      |      -6596 , -6201 , -5805 , -5409 , -5011 , ...
      |      -4613 , -4214 , -3815 , -3415 , -3014 , ...
      |      -2613 , -2212 , -1810 , -1408 , -1006 , ...
      |       -603 ,  -201 ...
      |     ])
  Sin3 : Lookup_n-D  Commented=on  NumberOfTableDimensions=1  BreakpointsSpecification=Even spacing  BreakpointsForDimension1=uint16(linspace(0,511,512))  BreakpointsForDimension1DataTypeStr=uint16  IndexSearchMethod=Linear search  BeginIndexSearchUsingPreviousIndexResult=on  UseOneInputPortForAllInputData=on  Table=int16(32767*sin(linspace(0,2*pi,512)))  TableDataTypeStr=int16  IntermediateResultsDataTypeStr=int32  InterpMethod=Flat  ExtrapMethod=Clip  RemoveProtectionInput=on  ApplyFullPrecisionForLinearInterpolation=on  InternalRulePriority=Speed  OutDataTypeStr=int16  RndMeth=Zero  FractionDataTypeStr=fixdt(1,16,0)  InputSameDT=off
  Sum1 : Sum  Inputs=|++
  Sum2 : Sum  Inputs=|++
  theta1 : InportShadow
  cos : Outport
  sin : Outport  Port=2
  wires:
  Shift Arithmetic/1 -> Sin1/1
  Sum2/1 -> Shift Arithmetic/1
  Constant3/1 -> Sum2/2
  Shift Arithmetic1/1 -> Sin/1
  theta1/1 -> Sum2/1
  theta/1 -> Sum1/1
  Sin/1 -> sin/1
  Sin1/1 -> cos/1
  Sum1/1 -> Shift Arithmetic1/1
  Constant1/1 -> Sum1/2

== system Senorless/FOC_PointModel/Observers/PLL/积分器 ==
  input : Inport
  Constant : Constant  OutDataTypeStr=int16
  Data Store Read1 : DataStoreRead  DataStoreName=Ts_Point  IndexOptions=Index vector (dialog)  Indices=1  OutputSizes=1
  Data Type Conversion3 : DataTypeConversion  Commented=on  OutDataTypeStr=int16  SaturateOnIntegerOverflow=off
  Divide : Product  Commented=on  Inputs=*/  OutDataTypeStr=int32  RndMeth=Zero
  Product1 : Product  OutDataTypeStr=int32  RndMeth=Zero
  Product2 : Product  OutDataTypeStr=int32  RndMeth=Zero
  Shift Arithmetic : ArithShift  BitShiftNumberSource=Input port  BitShiftNumber=8  BitShiftDirection=Right
      settings: InputPortMap=u0,p1
  Sum : Sum  Inputs=|++  OutDataTypeStr=int32  RndMeth=Zero
  Sum1 : Sum  Inputs=|++  OutDataTypeStr=int32  RndMeth=Zero
  Ts适当放大的缩小系数， 详见初始化模块 : ArithShift  Commented=on  BitShiftNumber=TS_POINT_GAIN  DiagnosticForOORShift=Error
  Unit Delay : UnitDelay  SampleTime=-1  HasFrameUpgradeWarning=on
  周期定点化适当放大2^n : Constant  Value=TS_POINT_GAIN
  积分器运行频率 : Constant  Commented=on  Value=FOC_FRQ
  这个是缩小周期增益的 : ArithShift  BitShiftNumber=15  DiagnosticForOORShift=Error
  output : Outport
  wires:
  积分器运行频率/1 -> Data Type Conversion3/1
  Data Type Conversion3/1 -> Divide/2
  周期定点化适当放大2^n/1 -> Shift Arithmetic/2
  Unit Delay/1 -> Sum/2
  Shift Arithmetic/1 -> Product2/2
  Data Store Read1/1 -> Product2/1
  Product2/1 -> 这个是缩小周期增益的/1
  这个是缩小周期增益的/1 -> Sum1/2, Product1/2
  Constant/1 -> Product1/1
  Product1/1 -> Sum/1
  Sum/1 -> Sum1/1, Unit Delay/1
  Sum1/1 -> output/1
  input/1 -> Shift Arithmetic/1

== system Senorless/FOC_PointModel/Observers/PLL2/LPF ==
  note: y(n)=ax(n)+(1−a)y(n−1)
  note: a =(ω c​ T s​ )/(1+ω c​ T s​ )
  input : Inport
  Constant1 : Constant  Value=8  OutDataTypeStr=int16
  Constant5 : Constant  OutDataTypeStr=int16
  Product10 : Product  OutDataTypeStr=int32
  Product11 : Product  OutDataTypeStr=int32  RndMeth=Zero
  Saturation : Saturate  UpperLimit=15  LowerLimit=0  RndMeth=Zero
  Shift Arithmetic1 : ArithShift  BitShiftNumber=-4
  Shift Arithmetic9 : ArithShift  BitShiftNumber=4
  Sum10 : Sum  Inputs=-+
  Sum11 : Sum  OutDataTypeStr=int32  RndMeth=Zero
  Unit Delay9 : UnitDelay  SampleTime=-1  HasFrameUpgradeWarning=on
  output : Outport
  wires:
  Saturation/1 -> Product11/2, Sum10/1
  input/1 -> Product10/2
  Unit Delay9/1 -> Product11/1
  Product10/1 -> Sum11/2
  Product11/1 -> Sum11/1
  Sum10/1 -> Product10/1
  Shift Arithmetic1/1 -> Sum10/2
  Shift Arithmetic9/1 -> Unit Delay9/1, output/1
  Sum11/1 -> Shift Arithmetic9/1
  Constant5/1 -> Shift Arithmetic1/1
  Constant1/1 -> Saturation/1

== system Senorless/FOC_PointModel/Observers/PLL2/PI Controller ==
  input : Inport
  Kp : Inport  Port=2
  Ki : Inport  Port=3
  Data Store Read3 : DataStoreRead  DataStoreName=PLL_Limit  IndexOptions=Index vector (dialog)  Indices=1  OutputSizes=1
  Gain : Gain  Gain=-1  OutDataTypeStr=int32  RndMeth=Zero
  Product2 : Product  OutDataTypeStr=int32  RndMeth=Zero
  Saturation Dynamic2 : simulink/Discontinuities/Saturation Dynamic  OutMin=[]  OutMax=[]  OutDataTypeStr=Inherit: Same as second input  OutDataType=fixdt(1, 16)  OutScaling=2^-10  RndMeth=Zero  DoSatur=off
  Scope : Scope  NumInputPorts=2
  Sum : Sum  OutDataTypeStr=int32  RndMeth=Zero
  input1 : InportShadow
  积分器 : Subsystem
      settings: MinAlgLoopOccurrences=on
  output : Outport
  wires:
  [Limit] -> Saturation Dynamic2/1
  Sum/1 -> Saturation Dynamic2/2
  Gain/1 -> Saturation Dynamic2/3
  [Limit] -> Gain/1
  Data Store Read3/1 -> [Limit]
  Saturation Dynamic2/1 -> output/1
  积分器/1(output) -> Sum/2, Scope/2
  Product2/1 -> Scope/1, Sum/1
  input1/1 -> 积分器/2(input)
  Ki/1 -> 积分器/1(Ki)
  Kp/1 -> Product2/2
  input/1 -> Product2/1

== system Senorless/FOC_PointModel/Observers/PLL2/PLL_LPF1 ==
  note: a =(ω c​ T s​ )/(1+ω c​ T s​ )
  note: y(n)=ax(n)+(1−a)y(n−1)
  input : Inport
  Constant1 : Constant  Value=PLL_LPF_LEVEL  OutDataTypeStr=int16
  Constant5 : Constant  OutDataTypeStr=int16
  Product10 : Product  OutDataTypeStr=int32
  Product11 : Product  OutDataTypeStr=int32  RndMeth=Zero
  Shift Arithmetic1 : ArithShift  BitShiftNumber=-4
  Shift Arithmetic9 : ArithShift  BitShiftNumber=4
  Sum10 : Sum  Inputs=-+
  Sum11 : Sum  OutDataTypeStr=int32  RndMeth=Zero
  Unit Delay9 : UnitDelay  SampleTime=-1  HasFrameUpgradeWarning=on
  output : Outport
  wires:
  Constant1/1 -> Sum10/1, Product11/2
  Constant5/1 -> Shift Arithmetic1/1
  Sum11/1 -> Shift Arithmetic9/1
  Shift Arithmetic9/1 -> output/1, Unit Delay9/1
  Shift Arithmetic1/1 -> Sum10/2
  Sum10/1 -> Product10/1
  Product11/1 -> Sum11/1
  Product10/1 -> Sum11/2
  Unit Delay9/1 -> Product11/1
  input/1 -> Product10/2

== system Senorless/FOC_PointModel/Observers/PLL2/sincos_512 ==
  theta : Inport
  Constant3 : Constant  Value=16384  OutDataTypeStr=uint16
  Shift Arithmetic : ArithShift  BitShiftNumber=7
  Shift Arithmetic1 : ArithShift  BitShiftNumber=7
  Sin : Lookup_n-D  NumberOfTableDimensions=1  BreakpointsSpecification=Even spacing  BreakpointsForDimension1=uint16(linspace(0,511,512))  BreakpointsForDimension1DataTypeStr=uint16  IndexSearchMethod=Linear search  BeginIndexSearchUsingPreviousIndexResult=on  UseOneInputPortForAllInputData=on  Table=int16(32767*sin(linspace(0,2*pi,512)))  TableDataTypeStr=int16  IntermediateResultsDataTypeStr=int32  InterpMethod=Flat  ExtrapMethod=Clip  RemoveProtectionInput=on  ApplyFullPrecisionForLinearInterpolation=on  InternalRulePriority=Speed  OutDataTypeStr=int16  RndMeth=Zero  FractionDataTypeStr=fixdt(1,16,0)  InputSameDT=off
  Sin1 : Lookup_n-D  NumberOfTableDimensions=1  BreakpointsSpecification=Even spacing  BreakpointsForDimension1=uint16(linspace(0,511,512))  BreakpointsForDimension1DataTypeStr=uint16  IndexSearchMethod=Linear search  BeginIndexSearchUsingPreviousIndexResult=on  UseOneInputPortForAllInputData=on  Table=int16(32767*sin(linspace(0,2*pi,512)))  TableDataTypeStr=int16  IntermediateResultsDataTypeStr=int32  InterpMethod=Flat  ExtrapMethod=Clip  RemoveProtectionInput=on  ApplyFullPrecisionForLinearInterpolation=on  InternalRulePriority=Speed  OutDataTypeStr=int16  RndMeth=Zero  FractionDataTypeStr=fixdt(1,16,0)  InputSameDT=off
  Sum2 : Sum  Inputs=|++
  theta1 : InportShadow
  cos : Outport
  sin : Outport  Port=2
  wires:
  theta/1 -> Shift Arithmetic1/1
  theta1/1 -> Sum2/1
  Shift Arithmetic1/1 -> Sin/1
  Constant3/1 -> Sum2/2
  Sum2/1 -> Shift Arithmetic/1
  Shift Arithmetic/1 -> Sin1/1
  Sin/1 -> sin/1
  Sin1/1 -> cos/1

== system Senorless/FOC_PointModel/Observers/PLL2/积分器 ==
  input : Inport
  Constant : Constant  OutDataTypeStr=int16
  Data Store Read1 : DataStoreRead  DataStoreName=Ts_Point  IndexOptions=Index vector (dialog)  Indices=1  OutputSizes=1
  Data Type Conversion3 : DataTypeConversion  Commented=on  OutDataTypeStr=int16  SaturateOnIntegerOverflow=off
  Divide : Product  Commented=on  Inputs=*/  OutDataTypeStr=int32  RndMeth=Zero
  Product1 : Product  OutDataTypeStr=int32  RndMeth=Zero
  Product2 : Product  OutDataTypeStr=int32  RndMeth=Zero
  Shift Arithmetic : ArithShift  BitShiftNumberSource=Input port  BitShiftNumber=8  BitShiftDirection=Right
      settings: InputPortMap=u0,p1
  Sum : Sum  Inputs=|++  OutDataTypeStr=int32  RndMeth=Zero
  Ts适当放大的缩小系数， 详见初始化模块 : ArithShift  Commented=on  BitShiftNumber=TS_POINT_GAIN  DiagnosticForOORShift=Error
  Unit Delay : UnitDelay  SampleTime=-1  HasFrameUpgradeWarning=on
  周期定点化适当放大2^n : Constant  Value=TS_POINT_GAIN
  积分器运行频率 : Constant  Commented=on  Value=FOC_FRQ
  这个是缩小周期增益的 : ArithShift  BitShiftNumber=15  DiagnosticForOORShift=Error
  output : Outport
  wires:
  Product1/1 -> Sum/1
  Constant/1 -> Product1/1
  这个是缩小周期增益的/1 -> Product1/2
  Product2/1 -> 这个是缩小周期增益的/1
  Data Store Read1/1 -> Product2/1
  Shift Arithmetic/1 -> Product2/2
  input/1 -> Shift Arithmetic/1
  Unit Delay/1 -> Sum/2
  Sum/1 -> Unit Delay/1, output/1
  周期定点化适当放大2^n/1 -> Shift Arithmetic/2
  Data Type Conversion3/1 -> Divide/2
  积分器运行频率/1 -> Data Type Conversion3/1
